simulink model "Model_TranslationEngine64"  (R2022b)
settings: Solver=FixedStepDiscrete  StartTime=0.0  StopTime=5  RelTol=1e-3  EnableMultiTasking=on
InitFcn:
  | % Initialize model
  | ModelSettings=BTConfig.GetModelSettings();
  | 
  | ModelSettings.Validate();
  | 
  | ModelInit;
  | 
  | 
  | % load library data
  | GainLibrary_data;
  | % Load saved values from partition process
  | CapturedConstMask.LoadMapFromFile(bdroot)
StartFcn:
  | % make sure all the simulated RTC requests are found
  | %RTC_SIM_OBJ.ValidateREQs();
undefined symbols (not defined in the file or in its folder): AA, BPLP, Column, NumHFRefBPF, NumHFRefLPF, NumMusicChannels, Row, VolumeMuteConfig
libraries: TuneVar x925, TOP x490, FeaturePath x111, CapturedConstLib x52
(part 4 of 34)

== system Model_TranslationEngine64/NEAR/Near1p1/VolumeMute/VolMuteCh1 ==
  Ann1NonEntGainCalc : Subsystem  mask(Blocklib NonEntGainCalc){Config=Config.Ann1NonEntGainCalc, FeatureName=Ann1NonEntGainCalc}
      mask prompts: Config "NonEntGainCalcConfig"; FeatureName "Feature path name:"
      mask init:
      | blkh=gcbh;
      | Config=BTConfig.Assert(blkh,Config);
      | 
      | Config.Validate();
      | BTConfig.InitSetFeatureIfPresent(blkh,'FeatureName');
      | 
      | % Flatten for MFB is not needed due to mask on MFB. Nice.
      mask Callback Config: BTConfig.CallbackHideIfPresent(gcbh,{'FeatureName'});
      mask TypeOptions FeatureName: FeaturePath/FeatureName
      mask DialogControl ParameterGroupVar2 Prompt: OverRides
  Ann1NonEntVncApplied : Subsystem  mask(Blocklib NonEntVncApplied){Config=Config.Ann1NonEntVncApplied, FeatureName=Ann1NonEntVncApplied}
      mask prompts: Config "NonEntVncAppliedConfig"; FeatureName "Feature path name:"
      mask init:
      | blkh=gcbh;
      | Config=BTConfig.Assert(blkh,Config);
      | Config.Validate();
      | BTConfig.InitSetFeatureIfPresent(blkh,'FeatureName');
      mask Callback Config: BTConfig.CallbackHideIfPresent(gcbh,{'FeatureName'});
      mask TypeOptions FeatureName: FeaturePath/FeatureName
  FeaturePath : FeaturePath/FeaturePath  FeatureName=Ann1  IsGroup=off  GroupNumber=-1  IsModule=off  TriggerInit=[270 -291 385 -184]
      settings: SourceProductName=Bose Talaria
  Mute : Subsystem  mask(Blocklib Mute){Config=Config.Ann1Mute, FeatureName=Ann1Mute}
      mask prompts: Config "MuteConfig"; FeatureName "Feature path name:"
      mask help: This block offers a simple mute feature using rgainy block. Set initial mute state for system cold start and a feature path name as desired. There are no tunable components, but runtime control is included.
      mask init:
      | blkh=gcbh;
      | Config=BTConfig.Assert(blkh,Config);
      | BTConfig.InitSetFeatureIfPresent(blkh,'FeatureName');
      | Config.Validate();
      mask Help:
      | This block offers a simple mute feature using rgainy block. The initial mute status of the block can be set through the mask.
      | 
      | RTC CONTROL:
      | Run time control is available to dynamically mute the audio. The mute status can be provided ('1' to mute audio), along with a ramp time and rate (rate gets precedence).
      | RTC_SIM_OBJ.AddREQ( 'MuteSet', 0.6, [0005,  <mute_status>, <ramp_db_per_second>, <ramp_time>]);
      | E.g., RTC_SIM_OBJ.AddREQ( 'MuteSet', 0.7, [0002, 1, 0, 50]);
      mask Callback Config: BTConfig.CallbackHideIfPresent(gcbh,{'FeatureName'});
      mask TypeOptions FeatureName: MuteControl/FeatureName
      mask Display:
      | [path,w,h] = IconMuteMask();
      | 
      | % work in pixels since the icon does not scale
      | pos = get(gcbh,'position');
      | bw = pos(3) - pos(1);
      | bh = pos(4) - pos(2);
      | 
      | % Draw centered icon
      | xAdj = bw/2 - w/2;
      | yAdj = bh/2 - h/2;
      | for i=1:length(path)
      |     if (path(i).rgb(1) >= 0)
      |         patch(path(i).x+xAdj, path(i).y+yAdj, path(i).rgb);
      |     end
      |     if (path(i).stroke(1) >= 0)
      |         plot(path(i).x+xAdj, path(i).y+yAdj);
      |     end
      | end
      | 
      | % Display some text
      | text(bw/2, 2,FeatureName, ...
      |     'horizontalAlignment','center', ...
      |     'VerticalAlignment','bottom');
  Volume : Subsystem  mask(Blocklib AnnVolume){FeatureName=Ann1Volume, Config=Config.Ann1Volume, TriggerInit=[50 25 130 85]}
      mask prompts: FeatureName "Feature path name:"; Config "AnnVolumeConfig"; TriggerInit "Hidden: MoveFcn redraw"
      mask help: This volume signal block includes receipt of volume level (via RTC) as well as tuning variables to calibrate a gain table that maps 8-bit integer volume index (from RTC) to float decibels.
      mask init:
      | blkh=gcbh;
      | Config=BTConfig.Assert(blkh,Config);
      | BTConfig.InitSetFeatureIfPresent(blkh,'FeatureName');
      | Config.Validate();
      settings: MoveFcn=VolumeMask.CB_TriggerInit(gcbh);
      mask TypeOptions FeatureName: FeaturePath/FeatureName
      mask Callback Config: BTConfig.CallbackHideIfPresent(gcbh,{'FeatureName'});
      mask Callback TriggerInit: VolumeMask.CB_TriggerInit(gcbh);
      mask Display:
      | [path,w,h] = IconVolumeMask();
      | 
      | % work in pixels since the icon does not scale
      | pos = get(gcbh,'position');
      | bw = pos(3) - pos(1);
      | bh = pos(4) - pos(2);
      | 
      | % Draw centered icon
      | xAdj = bw/2 - w/2;
      | yAdj = bh/2 - h/2;
      | for i=1:length(path)
      |     if (path(i).rgb(1) >= 0)
      |         patch(path(i).x+xAdj, path(i).y+yAdj, path(i).rgb);
      |     end
      |     if (path(i).stroke(1) >= 0)
      |         plot(path(i).x+xAdj, path(i).y+yAdj);
      |     end
      | end
      | 
      | % Display some text
      | text(bw/2, bh/2,FeatureName, ...
      |     'horizontalAlignment','center', ...
      |     'VerticalAlignment','middle');

== system Model_TranslationEngine64/NEAR/Near1p1/VolumeMute/VolMuteCh2 ==
  Ann2NonEntGainCalc : Subsystem  mask(Blocklib NonEntGainCalc){Config=Config.Ann2NonEntGainCalc, FeatureName=Ann2NonEntGainCalc}
      mask prompts: Config "NonEntGainCalcConfig"; FeatureName "Feature path name:"
      mask init:
      | blkh=gcbh;
      | Config=BTConfig.Assert(blkh,Config);
      | 
      | Config.Validate();
      | BTConfig.InitSetFeatureIfPresent(blkh,'FeatureName');
      | 
      | % Flatten for MFB is not needed due to mask on MFB. Nice.
      mask Callback Config: BTConfig.CallbackHideIfPresent(gcbh,{'FeatureName'});
      mask TypeOptions FeatureName: FeaturePath/FeatureName
      mask DialogControl ParameterGroupVar2 Prompt: OverRides
  Ann2NonEntVncApplied : Subsystem  mask(Blocklib NonEntVncApplied){Config=Config.Ann2NonEntVncApplied, FeatureName=Ann2NonEntVncApplied}
      mask prompts: Config "NonEntVncAppliedConfig"; FeatureName "Feature path name:"
      mask init:
      | blkh=gcbh;
      | Config=BTConfig.Assert(blkh,Config);
      | Config.Validate();
      | BTConfig.InitSetFeatureIfPresent(blkh,'FeatureName');
      mask Callback Config: BTConfig.CallbackHideIfPresent(gcbh,{'FeatureName'});
      mask TypeOptions FeatureName: FeaturePath/FeatureName
  FeaturePath : FeaturePath/FeaturePath  FeatureName=Ann2  IsGroup=off  GroupNumber=-1  IsModule=off  TriggerInit=[60 -206 175 -99]
      settings: SourceProductName=Bose Talaria
  Mute : Subsystem  mask(Blocklib Mute){Config=Config.Ann2Mute, FeatureName=Ann2Mute}
      mask prompts: Config "MuteConfig"; FeatureName "Feature path name:"
      mask help: This block offers a simple mute feature using rgainy block. Set initial mute state for system cold start and a feature path name as desired. There are no tunable components, but runtime control is included.
      mask init:
      | blkh=gcbh;
      | Config=BTConfig.Assert(blkh,Config);
      | BTConfig.InitSetFeatureIfPresent(blkh,'FeatureName');
      | Config.Validate();
      mask Help:
      | This block offers a simple mute feature using rgainy block. The initial mute status of the block can be set through the mask.
      | 
      | RTC CONTROL:
      | Run time control is available to dynamically mute the audio. The mute status can be provided ('1' to mute audio), along with a ramp time and rate (rate gets precedence).
      | RTC_SIM_OBJ.AddREQ( 'MuteSet', 0.6, [0005,  <mute_status>, <ramp_db_per_second>, <ramp_time>]);
      | E.g., RTC_SIM_OBJ.AddREQ( 'MuteSet', 0.7, [0002, 1, 0, 50]);
      mask Callback Config: BTConfig.CallbackHideIfPresent(gcbh,{'FeatureName'});
      mask TypeOptions FeatureName: MuteControl/FeatureName
      mask Display:
      | [path,w,h] = IconMuteMask();
      | 
      | % work in pixels since the icon does not scale
      | pos = get(gcbh,'position');
      | bw = pos(3) - pos(1);
      | bh = pos(4) - pos(2);
      | 
      | % Draw centered icon
      | xAdj = bw/2 - w/2;
      | yAdj = bh/2 - h/2;
      | for i=1:length(path)
      |     if (path(i).rgb(1) >= 0)
      |         patch(path(i).x+xAdj, path(i).y+yAdj, path(i).rgb);
      |     end
      |     if (path(i).stroke(1) >= 0)
      |         plot(path(i).x+xAdj, path(i).y+yAdj);
      |     end
      | end
      | 
      | % Display some text
      | text(bw/2, 2,FeatureName, ...
      |     'horizontalAlignment','center', ...
      |     'VerticalAlignment','bottom');
  Volume : Subsystem  mask(Blocklib AnnVolume){FeatureName=Ann2Volume, Config=Config.Ann2Volume, TriggerInit=[0 -25 80 35]}
      mask prompts: FeatureName "Feature path name:"; Config "AnnVolumeConfig"; TriggerInit "Hidden: MoveFcn redraw"
      mask help: This volume signal block includes receipt of volume level (via RTC) as well as tuning variables to calibrate a gain table that maps 8-bit integer volume index (from RTC) to float decibels.
      mask init:
      | blkh=gcbh;
      | Config=BTConfig.Assert(blkh,Config);
      | BTConfig.InitSetFeatureIfPresent(blkh,'FeatureName');
      | Config.Validate();
      settings: MoveFcn=VolumeMask.CB_TriggerInit(gcbh);
      mask TypeOptions FeatureName: FeaturePath/FeatureName
      mask Callback Config: BTConfig.CallbackHideIfPresent(gcbh,{'FeatureName'});
      mask Callback TriggerInit: VolumeMask.CB_TriggerInit(gcbh);
      mask Display:
      | [path,w,h] = IconVolumeMask();
      | 
      | % work in pixels since the icon does not scale
      | pos = get(gcbh,'position');
      | bw = pos(3) - pos(1);
      | bh = pos(4) - pos(2);
      | 
      | % Draw centered icon
      | xAdj = bw/2 - w/2;
      | yAdj = bh/2 - h/2;
      | for i=1:length(path)
      |     if (path(i).rgb(1) >= 0)
      |         patch(path(i).x+xAdj, path(i).y+yAdj, path(i).rgb);
      |     end
      |     if (path(i).stroke(1) >= 0)
      |         plot(path(i).x+xAdj, path(i).y+yAdj);
      |     end
      | end
      | 
      | % Display some text
      | text(bw/2, bh/2,FeatureName, ...
      |     'horizontalAlignment','center', ...
      |     'VerticalAlignment','middle');

== system Model_TranslationEngine64/NEAR/Near1p1/VolumeMute/VolMuteCh3 ==
  Ann3NonEntGainCalc : Subsystem  mask(Blocklib NonEntGainCalc){Config=Config.Ann3NonEntGainCalc, FeatureName=Ann3NonEntGainCalc}
      mask prompts: Config "NonEntGainCalcConfig"; FeatureName "Feature path name:"
      mask init:
      | blkh=gcbh;
      | Config=BTConfig.Assert(blkh,Config);
      | 
      | Config.Validate();
      | BTConfig.InitSetFeatureIfPresent(blkh,'FeatureName');
      | 
      | % Flatten for MFB is not needed due to mask on MFB. Nice.
      mask Callback Config: BTConfig.CallbackHideIfPresent(gcbh,{'FeatureName'});
      mask TypeOptions FeatureName: FeaturePath/FeatureName
      mask DialogControl ParameterGroupVar2 Prompt: OverRides
  Ann3NonEntVncApplied : Subsystem  mask(Blocklib NonEntVncApplied){Config=Config.Ann3NonEntVncApplied, FeatureName=Ann3NonEntVncApplied}
      mask prompts: Config "NonEntVncAppliedConfig"; FeatureName "Feature path name:"
      mask init:
      | blkh=gcbh;
      | Config=BTConfig.Assert(blkh,Config);
      | Config.Validate();
      | BTConfig.InitSetFeatureIfPresent(blkh,'FeatureName');
      mask Callback Config: BTConfig.CallbackHideIfPresent(gcbh,{'FeatureName'});
      mask TypeOptions FeatureName: FeaturePath/FeatureName
  FeaturePath : FeaturePath/FeaturePath  FeatureName=Ann3  IsGroup=off  GroupNumber=-1  IsModule=off  TriggerInit=[265 -336 380 -229]
      settings: SourceProductName=Bose Talaria
  Mute : Subsystem  mask(Blocklib Mute){Config=Config.Ann3Mute, FeatureName=Ann3Mute}
      mask prompts: Config "MuteConfig"; FeatureName "Feature path name:"
      mask help: This block offers a simple mute feature using rgainy block. Set initial mute state for system cold start and a feature path name as desired. There are no tunable components, but runtime control is included.
      mask init:
      | blkh=gcbh;
      | Config=BTConfig.Assert(blkh,Config);
      | BTConfig.InitSetFeatureIfPresent(blkh,'FeatureName');
      | Config.Validate();
      mask Help:
      | This block offers a simple mute feature using rgainy block. The initial mute status of the block can be set through the mask.
      | 
      | RTC CONTROL:
      | Run time control is available to dynamically mute the audio. The mute status can be provided ('1' to mute audio), along with a ramp time and rate (rate gets precedence).
      | RTC_SIM_OBJ.AddREQ( 'MuteSet', 0.6, [0005,  <mute_status>, <ramp_db_per_second>, <ramp_time>]);
      | E.g., RTC_SIM_OBJ.AddREQ( 'MuteSet', 0.7, [0002, 1, 0, 50]);
      mask Callback Config: BTConfig.CallbackHideIfPresent(gcbh,{'FeatureName'});
      mask TypeOptions FeatureName: MuteControl/FeatureName
      mask Display:
      | [path,w,h] = IconMuteMask();
      | 
      | % work in pixels since the icon does not scale
      | pos = get(gcbh,'position');
      | bw = pos(3) - pos(1);
      | bh = pos(4) - pos(2);
      | 
      | % Draw centered icon
      | xAdj = bw/2 - w/2;
      | yAdj = bh/2 - h/2;
      | for i=1:length(path)
      |     if (path(i).rgb(1) >= 0)
      |         patch(path(i).x+xAdj, path(i).y+yAdj, path(i).rgb);
      |     end
      |     if (path(i).stroke(1) >= 0)
      |         plot(path(i).x+xAdj, path(i).y+yAdj);
      |     end
      | end
      | 
      | % Display some text
      | text(bw/2, 2,FeatureName, ...
      |     'horizontalAlignment','center', ...
      |     'VerticalAlignment','bottom');
  Volume : Subsystem  mask(Blocklib AnnVolume){FeatureName=Ann3Volume, Config=Config.Ann3Volume, TriggerInit=[815 415 895 475]}
      mask prompts: FeatureName "Feature path name:"; Config "AnnVolumeConfig"; TriggerInit "Hidden: MoveFcn redraw"
      mask help: This volume signal block includes receipt of volume level (via RTC) as well as tuning variables to calibrate a gain table that maps 8-bit integer volume index (from RTC) to float decibels.
      mask init:
      | blkh=gcbh;
      | Config=BTConfig.Assert(blkh,Config);
      | BTConfig.InitSetFeatureIfPresent(blkh,'FeatureName');
      | Config.Validate();
      settings: MoveFcn=VolumeMask.CB_TriggerInit(gcbh);
      mask TypeOptions FeatureName: FeaturePath/FeatureName
      mask Callback Config: BTConfig.CallbackHideIfPresent(gcbh,{'FeatureName'});
      mask Callback TriggerInit: VolumeMask.CB_TriggerInit(gcbh);
      mask Display:
      | [path,w,h] = IconVolumeMask();
      | 
      | % work in pixels since the icon does not scale
      | pos = get(gcbh,'position');
      | bw = pos(3) - pos(1);
      | bh = pos(4) - pos(2);
      | 
      | % Draw centered icon
      | xAdj = bw/2 - w/2;
      | yAdj = bh/2 - h/2;
      | for i=1:length(path)
      |     if (path(i).rgb(1) >= 0)
      |         patch(path(i).x+xAdj, path(i).y+yAdj, path(i).rgb);
      |     end
      |     if (path(i).stroke(1) >= 0)
      |         plot(path(i).x+xAdj, path(i).y+yAdj);
      |     end
      | end
      | 
      | % Display some text
      | text(bw/2, bh/2,FeatureName, ...
      |     'horizontalAlignment','center', ...
      |     'VerticalAlignment','middle');

== system Model_TranslationEngine64/NEAR/Near1p1/VolumeMute/VolMuteCh4 ==
  Ann4NonEntGainCalc : Subsystem  mask(Blocklib NonEntGainCalc){Config=Config.Ann4NonEntGainCalc, FeatureName=Ann4NonEntGainCalc}
      mask prompts: Config "NonEntGainCalcConfig"; FeatureName "Feature path name:"
      mask init:
      | blkh=gcbh;
      | Config=BTConfig.Assert(blkh,Config);
      | 
      | Config.Validate();
      | BTConfig.InitSetFeatureIfPresent(blkh,'FeatureName');
      | 
      | % Flatten for MFB is not needed due to mask on MFB. Nice.
      mask Callback Config: BTConfig.CallbackHideIfPresent(gcbh,{'FeatureName'});
      mask TypeOptions FeatureName: FeaturePath/FeatureName
      mask DialogControl ParameterGroupVar2 Prompt: OverRides
  Ann4NonEntVncApplied : Subsystem  mask(Blocklib NonEntVncApplied){Config=Config.Ann4NonEntVncApplied, FeatureName=Ann4NonEntVncApplied}
      mask prompts: Config "NonEntVncAppliedConfig"; FeatureName "Feature path name:"
      mask init:
      | blkh=gcbh;
      | Config=BTConfig.Assert(blkh,Config);
      | Config.Validate();
      | BTConfig.InitSetFeatureIfPresent(blkh,'FeatureName');
      mask Callback Config: BTConfig.CallbackHideIfPresent(gcbh,{'FeatureName'});
      mask TypeOptions FeatureName: FeaturePath/FeatureName
  FeaturePath : FeaturePath/FeaturePath  FeatureName=Ann4  IsGroup=off  GroupNumber=-1  IsModule=off  TriggerInit=[235 -186 350 -79]
      settings: SourceProductName=Bose Talaria
  Mute : Subsystem  mask(Blocklib Mute){Config=Config.Ann4Mute, FeatureName=Ann4Mute}
      mask prompts: Config "MuteConfig"; FeatureName "Feature path name:"
      mask help: This block offers a simple mute feature using rgainy block. Set initial mute state for system cold start and a feature path name as desired. There are no tunable components, but runtime control is included.
      mask init:
      | blkh=gcbh;
      | Config=BTConfig.Assert(blkh,Config);
      | BTConfig.InitSetFeatureIfPresent(blkh,'FeatureName');
      | Config.Validate();
      mask Help:
      | This block offers a simple mute feature using rgainy block. The initial mute status of the block can be set through the mask.
      | 
      | RTC CONTROL:
      | Run time control is available to dynamically mute the audio. The mute status can be provided ('1' to mute audio), along with a ramp time and rate (rate gets precedence).
      | RTC_SIM_OBJ.AddREQ( 'MuteSet', 0.6, [0005,  <mute_status>, <ramp_db_per_second>, <ramp_time>]);
      | E.g., RTC_SIM_OBJ.AddREQ( 'MuteSet', 0.7, [0002, 1, 0, 50]);
      mask Callback Config: BTConfig.CallbackHideIfPresent(gcbh,{'FeatureName'});
      mask TypeOptions FeatureName: MuteControl/FeatureName
      mask Display:
      | [path,w,h] = IconMuteMask();
      | 
      | % work in pixels since the icon does not scale
      | pos = get(gcbh,'position');
      | bw = pos(3) - pos(1);
      | bh = pos(4) - pos(2);
      | 
      | % Draw centered icon
      | xAdj = bw/2 - w/2;
      | yAdj = bh/2 - h/2;
      | for i=1:length(path)
      |     if (path(i).rgb(1) >= 0)
      |         patch(path(i).x+xAdj, path(i).y+yAdj, path(i).rgb);
      |     end
      |     if (path(i).stroke(1) >= 0)
      |         plot(path(i).x+xAdj, path(i).y+yAdj);
      |     end
      | end
      | 
      | % Display some text
      | text(bw/2, 2,FeatureName, ...
      |     'horizontalAlignment','center', ...
      |     'VerticalAlignment','bottom');
  Volume : Subsystem  mask(Blocklib AnnVolume){FeatureName=Ann4Volume, Config=Config.Ann4Volume, TriggerInit=[20 5 100 65]}
      mask prompts: FeatureName "Feature path name:"; Config "AnnVolumeConfig"; TriggerInit "Hidden: MoveFcn redraw"
      mask help: This volume signal block includes receipt of volume level (via RTC) as well as tuning variables to calibrate a gain table that maps 8-bit integer volume index (from RTC) to float decibels.
      mask init:
      | blkh=gcbh;
      | Config=BTConfig.Assert(blkh,Config);
      | BTConfig.InitSetFeatureIfPresent(blkh,'FeatureName');
      | Config.Validate();
      settings: MoveFcn=VolumeMask.CB_TriggerInit(gcbh);
      mask TypeOptions FeatureName: FeaturePath/FeatureName
      mask Callback Config: BTConfig.CallbackHideIfPresent(gcbh,{'FeatureName'});
      mask Callback TriggerInit: VolumeMask.CB_TriggerInit(gcbh);
      mask Display:
      | [path,w,h] = IconVolumeMask();
      | 
      | % work in pixels since the icon does not scale
      | pos = get(gcbh,'position');
      | bw = pos(3) - pos(1);
      | bh = pos(4) - pos(2);
      | 
      | % Draw centered icon
      | xAdj = bw/2 - w/2;
      | yAdj = bh/2 - h/2;
      | for i=1:length(path)
      |     if (path(i).rgb(1) >= 0)
      |         patch(path(i).x+xAdj, path(i).y+yAdj, path(i).rgb);
      |     end
      |     if (path(i).stroke(1) >= 0)
      |         plot(path(i).x+xAdj, path(i).y+yAdj);
      |     end
      | end
      | 
      | % Display some text
      | text(bw/2, bh/2,FeatureName, ...
      |     'horizontalAlignment','center', ...
      |     'VerticalAlignment','middle');

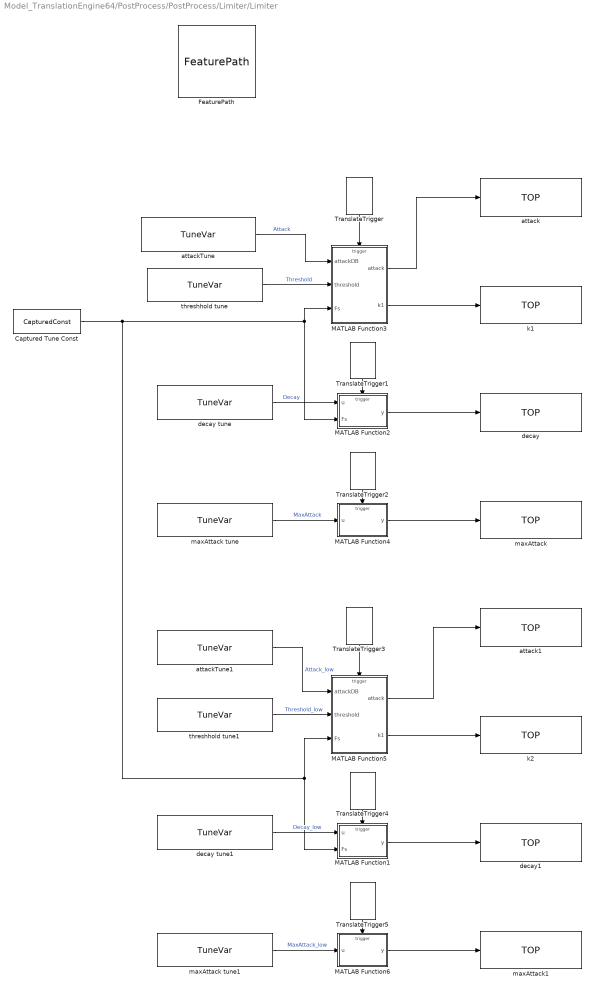
== system Model_TranslationEngine64/PostProcess/PostProcess/Limiter/Limiter ==
  Captured Tune Const : CapturedConstLib/CapturedConst  TriggerInit=[-235 487 -135 523]  Role=Automatic
      settings: SourceProductName=Bose Talaria
  FeaturePath : FeaturePath/FeaturePath  FeatureName=Limiter  IsGroup=off  GroupNumber=-1  IsModule=off  TriggerInit=[10 64 125 171]
      settings: SourceProductName=Bose Talaria
  MATLAB Function1 : MATLAB Function  TreatAsAtomicUnit=on
  MATLAB Function2 : MATLAB Function  TreatAsAtomicUnit=on
  MATLAB Function3 : MATLAB Function  TreatAsAtomicUnit=on
  MATLAB Function4 : MATLAB Function  TreatAsAtomicUnit=on
  MATLAB Function5 : MATLAB Function  TreatAsAtomicUnit=on
  MATLAB Function6 : MATLAB Function  TreatAsAtomicUnit=on
  TranslateTrigger : TuneVar/TranslateTrigger  TriggerInit=[261 290 299 345]
      settings: SourceProductName=Bose Talaria
  TranslateTrigger1 : TuneVar/TranslateTrigger  TriggerInit=[266 535 304 590]
      settings: SourceProductName=Bose Talaria
  TranslateTrigger2 : TuneVar/TranslateTrigger  TriggerInit=[266 700 304 755]
      settings: SourceProductName=Bose Talaria
  TranslateTrigger3 : TuneVar/TranslateTrigger  TriggerInit=[261 930 299 985]
      settings: SourceProductName=Bose Talaria
  TranslateTrigger4 : TuneVar/TranslateTrigger  TriggerInit=[266 1175 304 1230]
      settings: SourceProductName=Bose Talaria
  TranslateTrigger5 : TuneVar/TranslateTrigger  TriggerInit=[266 1340 304 1395]
      settings: SourceProductName=Bose Talaria
  attack : TOP/TOP  TriggerInit=[460 292 610 348]  TopName=attack  DataTypeOut=single  BankNumber=0  PreOverlay=false  PostOverlay=false  Role=Automatic
      settings: SourceProductName=Bose Talaria
  attack1 : TOP/TOP  TriggerInit=[460 932 610 988]  TopName=attack_low  DataTypeOut=single  BankNumber=0  PreOverlay=false  PostOverlay=false  Role=Automatic
      settings: SourceProductName=Bose Talaria
  attackTune : TuneVar/TuneVar  TuneName=Attack  SpecifyMaxSize=off  VariableDim=2 (Column)  MaxSize=[1 16]  TunabilityNumber=1  MinValue=[]  MaxValue=[]  TriggerInit=[-45 350 125 400]  MaskValue=Config.DefaultAttackDb
      settings: SourceProductName=Bose Talaria
  attackTune1 : TuneVar/TuneVar  TuneName=Attack_low  SpecifyMaxSize=off  VariableDim=2 (Column)  MaxSize=[1 1]  TunabilityNumber=1  MinValue=[]  MaxValue=[]  TriggerInit=[-20 965 150 1015]  MaskValue=Config.DefaultAttackLowDb
      settings: SourceProductName=Bose Talaria
  decay : TOP/TOP  TriggerInit=[460 612 610 668]  TopName=decay  DataTypeOut=single  BankNumber=0  PreOverlay=false  PostOverlay=false  Role=Automatic
      settings: SourceProductName=Bose Talaria
  decay tune : TuneVar/TuneVar  TuneName=Decay  SpecifyMaxSize=off  VariableDim=2 (Column)  MaxSize=[1 1]  TunabilityNumber=1  MinValue=[]  MaxValue=[]  TriggerInit=[-20 600 150 650]  MaskValue=Config.DefaultDecayDB
      settings: SourceProductName=Bose Talaria
  decay tune1 : TuneVar/TuneVar  TuneName=Decay_low  SpecifyMaxSize=off  VariableDim=2 (Column)  MaxSize=[1 1]  TunabilityNumber=1  MinValue=[]  MaxValue=[]  TriggerInit=[-20 1240 150 1290]  MaskValue=Config.DefaultDecayLowDb
      settings: SourceProductName=Bose Talaria
  decay1 : TOP/TOP  TriggerInit=[460 1252 610 1308]  TopName=decay_low  DataTypeOut=single  BankNumber=0  PreOverlay=false  PostOverlay=false  Role=Automatic
      settings: SourceProductName=Bose Talaria
  k1 : TOP/TOP  TriggerInit=[460 452 610 508]  TopName=k1  DataTypeOut=single  BankNumber=0  PreOverlay=false  PostOverlay=false  Role=Automatic
      settings: SourceProductName=Bose Talaria
  k2 : TOP/TOP  TriggerInit=[460 1092 610 1148]  TopName=k1_low  DataTypeOut=single  BankNumber=0  PreOverlay=false  PostOverlay=false  Role=Automatic
      settings: SourceProductName=Bose Talaria
  maxAttack : TOP/TOP  TriggerInit=[460 772 610 828]  TopName=maxAttack  DataTypeOut=single  BankNumber=0  PreOverlay=false  PostOverlay=false  Role=Automatic
      settings: SourceProductName=Bose Talaria
  maxAttack tune : TuneVar/TuneVar  TuneName=MaxAttack  SpecifyMaxSize=off  VariableDim=2 (Column)  MaxSize=[1 1]  TunabilityNumber=1  MinValue=[]  MaxValue=[]  TriggerInit=[-20 775 150 825]  MaskValue=Config.DefaultMaxAttackDb
      settings: SourceProductName=Bose Talaria
  maxAttack tune1 : TuneVar/TuneVar  TuneName=MaxAttack_low  SpecifyMaxSize=off  VariableDim=2 (Column)  MaxSize=[1 1]  TunabilityNumber=1  MinValue=[]  MaxValue=[]  TriggerInit=[-20 1415 150 1465]  MaskValue=Config.DefaultMaxAttackLowDb
      settings: SourceProductName=Bose Talaria
  maxAttack1 : TOP/TOP  TriggerInit=[460 1412 610 1468]  TopName=maxAttack_low  DataTypeOut=single  BankNumber=0  PreOverlay=false  PostOverlay=false  Role=Automatic
      settings: SourceProductName=Bose Talaria
  threshhold tune : TuneVar/TuneVar  TuneName=Threshold  SpecifyMaxSize=off  VariableDim=2 (Column)  MaxSize=[1 16]  TunabilityNumber=1  MinValue=[]  MaxValue=[]  TriggerInit=[-35 425 135 475]  MaskValue=Config.DefaultThreshold
      settings: SourceProductName=Bose Talaria
  threshhold tune1 : TuneVar/TuneVar  TuneName=Threshold_low  SpecifyMaxSize=off  VariableDim=2 (Column)  MaxSize=[1 1]  TunabilityNumber=1  MinValue=[]  MaxValue=[]  TriggerInit=[-20 1065 150 1115]  MaskValue=Config.DefaultThresholdLow
      settings: SourceProductName=Bose Talaria
  wires:
  TranslateTrigger4/1 -> MATLAB Function1/Trigger
  maxAttack tune1/1 -> MATLAB Function6/1(u)  "MaxAttack_low"
  TranslateTrigger3/1 -> MATLAB Function5/Trigger
  MATLAB Function5/2(k1) -> k2/1
  threshhold tune1/1 -> MATLAB Function5/2(threshold)  "Threshold_low"
  attackTune1/1 -> MATLAB Function5/1(attackDB)  "Attack_low"
  decay tune1/1 -> MATLAB Function1/1(u)  "Decay_low"
  MATLAB Function1/1(y) -> decay1/1
  Captured Tune Const/1 -> MATLAB Function1/2(Fs), MATLAB Function5/3(Fs), MATLAB Function2/2(Fs), MATLAB Function3/3(Fs)
  TranslateTrigger5/1 -> MATLAB Function6/Trigger
  MATLAB Function6/1(y) -> maxAttack1/1
  MATLAB Function5/1(attack) -> attack1/1
  MATLAB Function3/1(attack) -> attack/1
  MATLAB Function4/1(y) -> maxAttack/1
  TranslateTrigger2/1 -> MATLAB Function4/Trigger
  maxAttack tune/1 -> MATLAB Function4/1(u)  "MaxAttack"
  MATLAB Function3/2(k1) -> k1/1
  TranslateTrigger/1 -> MATLAB Function3/Trigger
  threshhold tune/1 -> MATLAB Function3/2(threshold)  "Threshold"
  MATLAB Function2/1(y) -> decay/1
  TranslateTrigger1/1 -> MATLAB Function2/Trigger
  decay tune/1 -> MATLAB Function2/1(u)  "Decay"
  attackTune/1 -> MATLAB Function3/1(attackDB)  "Attack"

== system Model_TranslationEngine64/PostProcess/PostProcess/Mute/Mute ==
  MuteControl : Subsystem  mask(Blocklib MuteControl){Config=Config, FeatureName=Mute}
      mask prompts: Config "MuteControlConfig"; FeatureName "Mask feature name:"
      mask help: This component is to be used in conjunction with 1 or more instances of the MuteRamper block. There is no mask for this component. It provides the control layer for Mute processing via an RTC and tune variable, muteControlRampTime.
      mask init:
      | blkh=gcbh;
      | Config=BTConfig.Assert(blkh,Config);
      | BTConfig.InitSetFeatureIfPresent(blkh,'FeatureName');
      | Config.Validate();
      | 
      | % Set boundary conditions
      | rampRateBounds = [5,50000];
      | rampTimeBounds = [1,3000];
      mask Help: If this control block is being used in a "multi-instance" manner, i.e. it is contorlling two or more MuteRamper blocks, there is an additional step that must be done. The developer must add a function-triggered subsytem containing an AND logic gate, which will combine the notification completion signals of the multiple ramper instances. The output of this subsytem must then feed the NTF_done input of the MuteControl block.
      mask Callback Config: BTConfig.CallbackHideIfPresent(gcbh,{'FeatureName'});
      mask TypeOptions FeatureName: FeaturePath/FeatureName

== system Model_TranslationEngine64/PostProcess/PostProcess/PostLimiterEQ/PoolIirTunableWithReset ==
  CapturedTuneConst : CapturedConstLib/CapturedConst  TriggerInit=[-600 302 -500 338]  Role=Automatic
      settings: SourceProductName=Bose Talaria
  FeaturePath : FeaturePath/FeaturePath  FeatureName=PostLimiterEq  IsGroup=off  GroupNumber=-1  IsModule=off  TriggerInit=[-750 -81 -635 26]
      settings: SourceProductName=Bose Talaria
  TOP : TOP/TOP  TriggerInit=[-145 187 5 243]  TopName=PooliirNumStages  DataTypeOut=uint32  BankNumber=0  PreOverlay=false  PostOverlay=Config.VariantObj.PostOverlayRequired  Role=Automatic
      settings: SourceProductName=Bose Talaria
  TOP1 : TOP/TOP  TriggerInit=[-140 277 10 333]  TopName=pooliirCoeffs  DataTypeOut=single  BankNumber=0  PreOverlay=false  PostOverlay=Config.VariantObj.PostOverlayRequired  Role=Automatic
      settings: SourceProductName=Bose Talaria
  TranslateTrigger : TuneVar/TranslateTrigger  TriggerInit=[-339 35 -301 90]
      settings: SourceProductName=Bose Talaria
  Translation : MATLAB Function  TreatAsAtomicUnit=on  mask{MaxNumStages=Config.MaxNumStages, VariantUint8=Config.Variant.Uint8Str}
      mask prompts: VariantUint8 "Variant"
  Tune Variable1 : TuneVar/TuneVar  TuneName=numStages  SpecifyMaxSize=off  VariableDim=1 (Row)  MaxSize=[1 1]  TunabilityNumber=1  MinValue=[]  MaxValue=[]  TriggerInit=[-750 235 -580 285]  MaskValue=Config.TuneDefaults.NumStages
      settings: SourceProductName=Bose Talaria
  Tune Variable2 : TuneVar/TuneVar  TuneName=sosCoefficients  SpecifyMaxSize=on  VariableDim=1 (Row)  MaxSize=[Config.MaxNumStages 6]  TunabilityNumber=1  MinValue=[]  MaxValue=[]  TriggerInit=[-750 175 -580 225]  MaskValue=Config.TuneDefaults.SosCoefficients
      settings: SourceProductName=Bose Talaria
  wires:
  CapturedTuneConst/1 -> Translation/3(NumChannels)
  Tune Variable1/1 -> Translation/2(NumStages)  "numStages"
  Translation/1(PoolNumStages) -> TOP/1
  Translation/2(PoolCoeffs) -> TOP1/1
  Tune Variable2/1 -> Translation/1(RawSOS)  "sosCoefficients"
  TranslateTrigger/1 -> Translation/Trigger

== system Model_TranslationEngine64/PostProcess/PostProcess/Soft Clipper/SoftClipper ==
  FeaturePath : FeaturePath/FeaturePath  FeatureName=SoftClipper  IsGroup=off  GroupNumber=-1  IsModule=off  TriggerInit=[-80 -61 25 36]
      settings: SourceProductName=Bose Talaria
  TranslateTrigger : TuneVar/TranslateTrigger  TriggerInit=[341 -20 379 35]
      settings: SourceProductName=Bose Talaria
  TranslateTrigger1 : TuneVar/TranslateTrigger  TriggerInit=[341 350 379 405]
      settings: SourceProductName=Bose Talaria
  p2 TOP : TOP/TOP  TriggerInit=[525 247 675 303]  TopName=p2  DataTypeOut=single  BankNumber=0  PreOverlay=false  PostOverlay=false  Role=Automatic
      settings: SourceProductName=Bose Talaria
  p2 TOP1 : TOP/TOP  TriggerInit=[525 587 675 643]  TopName=p2_low  DataTypeOut=single  BankNumber=0  PreOverlay=false  PostOverlay=false  Role=Automatic
      settings: SourceProductName=Bose Talaria
  translation : MATLAB Function  TreatAsAtomicUnit=on
  translation1 : MATLAB Function  TreatAsAtomicUnit=on
  xmax TOP : TOP/TOP  TriggerInit=[525 172 675 228]  TopName=xmax  DataTypeOut=single  BankNumber=0  PreOverlay=false  PostOverlay=false  Role=Automatic
      settings: SourceProductName=Bose Talaria
  xmax TOP1 : TOP/TOP  TriggerInit=[525 512 675 568]  TopName=xmax_low  DataTypeOut=single  BankNumber=0  PreOverlay=false  PostOverlay=false  Role=Automatic
      settings: SourceProductName=Bose Talaria
  xmin TOP : TOP/TOP  TriggerInit=[525 97 675 153]  TopName=xmin  DataTypeOut=single  BankNumber=0  PreOverlay=false  PostOverlay=false  Role=Automatic
      settings: SourceProductName=Bose Talaria
  xmin TOP1 : TOP/TOP  TriggerInit=[525 437 675 493]  TopName=xmin_low  DataTypeOut=single  BankNumber=0  PreOverlay=false  PostOverlay=false  Role=Automatic
      settings: SourceProductName=Bose Talaria
  xmin TuneVar : TuneVar/TuneVar  TuneName=XMin  SpecifyMaxSize=off  VariableDim=2 (Column)  MaxSize=[1 1]  TunabilityNumber=1  MinValue=[]  MaxValue=[]  TriggerInit=[20 230 190 280]  MaskValue=Config.DefaultXmin
      settings: SourceProductName=Bose Talaria
  xmin TuneVar1 : TuneVar/TuneVar  TuneName=XMinLow  SpecifyMaxSize=off  VariableDim=2 (Column)  MaxSize=[1 1]  TunabilityNumber=1  MinValue=[]  MaxValue=[]  TriggerInit=[20 570 190 620]  MaskValue=Config.DefaultXminLow
      settings: SourceProductName=Bose Talaria
  ymax TuneVar : TuneVar/TuneVar  TuneName=YMax  SpecifyMaxSize=off  VariableDim=2 (Column)  MaxSize=[1 1]  TunabilityNumber=1  MinValue=[]  MaxValue=[]  TriggerInit=[20 120 190 170]  MaskValue=Config.DefaultYmax
      settings: SourceProductName=Bose Talaria
  ymax TuneVar1 : TuneVar/TuneVar  TuneName=YMaxLow  SpecifyMaxSize=off  VariableDim=2 (Column)  MaxSize=[1 1]  TunabilityNumber=1  MinValue=[]  MaxValue=[]  TriggerInit=[20 460 190 510]  MaskValue=Config.DefaultYmaxLow
      settings: SourceProductName=Bose Talaria
  wires:
  translation1/2(xmax_top) -> xmax TOP1/1
  translation1/3(p2) -> p2 TOP1/1
  translation1/1(xmin_top) -> xmin TOP1/1
  xmin TuneVar1/1 -> translation1/2(xmin_tune)  "XMinLow"
  ymax TuneVar1/1 -> translation1/1(ymax_tune)  "YMaxLow"
  TranslateTrigger1/1 -> translation1/Trigger
  TranslateTrigger/1 -> translation/Trigger
  xmin TuneVar/1 -> translation/2(xmin_tune)  "XMin"
  ymax TuneVar/1 -> translation/1(ymax_tune)  "YMax"
  translation/3(p2) -> p2 TOP/1
  translation/2(xmax_top) -> xmax TOP/1
  translation/1(xmin_top) -> xmin TOP/1

== system Model_TranslationEngine64/TestRouter/ASDRouter/InnerLink/AuxChannel_with_MATLAB_function ==
  TuneTOP_enable_aux_flag : Subsystem  mask(Talaria Trivial Tune TOP){TriggerInit=[-445 144 -315 176], TopName=EnableAux, TuneName=EnableAux, DataTypeOut=int32, MaskValue=Config.EnableAux, TunabilityNumber=1, MinValue=[], MaxValue=[], BankNumber=0, PreOverlay=false, PostOverlay=false, UseSameName=on}
      mask prompts: TriggerInit "Hidden: MoveFcn redraw"; TopName "Name:"; TuneName "Name of TuneVar:"; DataTypeOut "Data type:"; MaskValue "Default Value:"; TunabilityNumber "Tunability:"; MinValue "Min Value:"; MaxValue "Max Value:"; BankNumber "Target memory bank number:"; PreOverlay "Requires pre-overlay action:"; PostOverlay "Requires post-overlay action:"; UseSameName "Use same name for tune variable and TOP"
      mask help: The TuneTOP block encapsultes a Target Overlay Parameter, a Tune Variable, and a Trivial Translation between them.
      mask init:
      | [ok,activeTopPath,activeTunePath] = TuneTOP_Mask.Init(gcbh);
      settings: MoveFcn=TuneTOP_Mask.CB_TriggerInit(gcbh);
      mask Callback TriggerInit: TuneTOP_Mask.CB_TriggerInit(gcbh);
      mask TypeOptions TopName: TOP/TopName
      mask TypeOptions TuneName: Tune Variable/TuneName
      mask TypeOptions DataTypeOut: TOP/DataTypeOut
      mask TypeOptions MaskValue: Tune Variable/MaskValue
      mask TypeOptions TunabilityNumber: Tune Variable/TunabilityNumber
      mask Callback TunabilityNumber: TuneVarMask.CB_TunabilityNumber(gcbh);
      mask TypeOptions MinValue: Tune Variable/MinValue
      mask TypeOptions MaxValue: Tune Variable/MaxValue
      mask TypeOptions BankNumber: TOP/BankNumber
      mask TypeOptions PreOverlay: TOP/PreOverlay
      mask TypeOptions PostOverlay: TOP/PostOverlay
      mask Callback UseSameName: TuneTOP_Mask.CB_UseSameName(gcbh);
      mask DialogControl toolPanel Prompt: Tuning Tool Hints
      mask DialogControl DescriptionGroup Prompt: Description
      mask DialogControl EditDescription Prompt: Edit Description
      mask DialogControl EditDescription Callback: TuneTOP_Mask.CB_EditDescription(gcbh);
      mask DialogControl TunabilityText Prompt: Easy: Changes nearly every tuning.
      mask DialogControl AdvancedPanel Prompt: Advanced
      mask DialogControl ConvertToFullTranslation Prompt: Irreversible conversion to full translation
      mask DialogControl ConvertToFullTranslation Callback: TuneTOP_Mask.CB_ConvertToFullTranslation(gcbh);
      mask DialogControl ErrorContainer Prompt: Error Messages
      mask DialogControl ErrorText Prompt: Default value cannot be empty. Tune variables must have non-zero dimensions.
      mask Display:
      | % retrieve icon definition
      | [path,w,h] = TuneTOP_Mask.Icon();
      | 
      | % retrieve the block's pixel size
      | pos = get(gcbh,'position');
      | bw = pos(3) - pos(1);
      | bh = pos(4) - pos(2);
      | 
      | % draw centered icon
      | xAdj = bw/2 - w/2 + 5;
      | yAdj = bh/2 - h/2 + 4;
      | for i=1:length(path)
      | 	patch(path(i).x+xAdj, path(i).y+yAdj, path(i).rgb);
      | end
      | 
      | % show the top name or an X
      | if (exist('ok','var') && ok)
      | 	text(bw*0.5, bh*0.2, activeTopPath, 'horizontalAlignment', 'center');
      | 	patch(0,0,[1 1 1]);
      | 	patch(bw,bh,[1 1 1]);
      | else
      | 	tx=bw*0.03;
      | 	ty=bh*0.03;
      | 	patch([0 tx bw bw-tx], [ty 0 bh-ty bh], [1 0 0]);
      | 	patch([0 bw-tx bw tx], [bh-ty 0 ty bh], [1 0 0]);
      | end

== system Model_TranslationEngine64/TestRouter/ASDRouter/InnerLink/MainChannelSystem ==
  TuneTOP_pmain_select : Subsystem  mask(Talaria Trivial Tune TOP){TriggerInit=[-390 156 -225 204], TopName=MainSelect, TuneName=MainSelect, DataTypeOut=int32, MaskValue=Config.MainSelect, TunabilityNumber=1, MinValue=[], MaxValue=[], BankNumber=0, PreOverlay=false, PostOverlay=false, UseSameName=on}
      mask prompts: TriggerInit "Hidden: MoveFcn redraw"; TopName "Name:"; TuneName "Name of TuneVar:"; DataTypeOut "Data type:"; MaskValue "Default Value:"; TunabilityNumber "Tunability:"; MinValue "Min Value:"; MaxValue "Max Value:"; BankNumber "Target memory bank number:"; PreOverlay "Requires pre-overlay action:"; PostOverlay "Requires post-overlay action:"; UseSameName "Use same name for tune variable and TOP"
      mask help: The TuneTOP block encapsultes a Target Overlay Parameter, a Tune Variable, and a Trivial Translation between them.
      mask init:
      | [ok,activeTopPath,activeTunePath] = TuneTOP_Mask.Init(gcbh);
      settings: MoveFcn=TuneTOP_Mask.CB_TriggerInit(gcbh);
      mask Callback TriggerInit: TuneTOP_Mask.CB_TriggerInit(gcbh);
      mask TypeOptions TopName: TOP/TopName
      mask TypeOptions TuneName: Tune Variable/TuneName
      mask TypeOptions DataTypeOut: TOP/DataTypeOut
      mask TypeOptions MaskValue: Tune Variable/MaskValue
      mask TypeOptions TunabilityNumber: Tune Variable/TunabilityNumber
      mask Callback TunabilityNumber: TuneVarMask.CB_TunabilityNumber(gcbh);
      mask TypeOptions MinValue: Tune Variable/MinValue
      mask TypeOptions MaxValue: Tune Variable/MaxValue
      mask TypeOptions BankNumber: TOP/BankNumber
      mask TypeOptions PreOverlay: TOP/PreOverlay
      mask TypeOptions PostOverlay: TOP/PostOverlay
      mask Callback UseSameName: TuneTOP_Mask.CB_UseSameName(gcbh);
      mask DialogControl toolPanel Prompt: Tuning Tool Hints
      mask DialogControl DescriptionGroup Prompt: Description
      mask DialogControl EditDescription Prompt: Edit Description
      mask DialogControl EditDescription Callback: TuneTOP_Mask.CB_EditDescription(gcbh);
      mask DialogControl TunabilityText Prompt: Easy: Changes nearly every tuning.
      mask DialogControl AdvancedPanel Prompt: Advanced
      mask DialogControl ConvertToFullTranslation Prompt: Irreversible conversion to full translation
      mask DialogControl ConvertToFullTranslation Callback: TuneTOP_Mask.CB_ConvertToFullTranslation(gcbh);
      mask DialogControl ErrorContainer Prompt: Error Messages
      mask DialogControl ErrorText Prompt: Default value cannot be empty. Tune variables must have non-zero dimensions.
      mask Display:
      | % retrieve icon definition
      | [path,w,h] = TuneTOP_Mask.Icon();
      | 
      | % retrieve the block's pixel size
      | pos = get(gcbh,'position');
      | bw = pos(3) - pos(1);
      | bh = pos(4) - pos(2);
      | 
      | % draw centered icon
      | xAdj = bw/2 - w/2 + 5;
      | yAdj = bh/2 - h/2 + 4;
      | for i=1:length(path)
      | 	patch(path(i).x+xAdj, path(i).y+yAdj, path(i).rgb);
      | end
      | 
      | % show the top name or an X
      | if (exist('ok','var') && ok)
      | 	text(bw*0.5, bh*0.2, activeTopPath, 'horizontalAlignment', 'center');
      | 	patch(0,0,[1 1 1]);
      | 	patch(bw,bh,[1 1 1]);
      | else
      | 	tx=bw*0.03;
      | 	ty=bh*0.03;
      | 	patch([0 tx bw bw-tx], [ty 0 bh-ty bh], [1 0 0]);
      | 	patch([0 bw-tx bw tx], [bh-ty 0 ty bh], [1 0 0]);
      | end

== system Model_TranslationEngine64/ModelPreAmp/DecRate/AudioPilot35/Audiopilot_3_5/ConfigurationRtcInputs ==
  note: Downgrade Flag
  note: HVAC
  note: Speed
  note: Mute
  AudiopilotTwoDowngrade : Subsystem  mask(Talaria Trivial Tune TOP){TriggerInit=[1655 1312 1805 1368], TopName=TwoDowngrade, TuneName=TwoDowngrade, DataTypeOut=uint32, MaskValue=0, TunabilityNumber=1, MinValue=[], MaxValue=[], BankNumber=0, PreOverlay=false, PostOverlay=false, UseSameName=on}
      mask prompts: TriggerInit "Hidden: MoveFcn redraw"; TopName "Name:"; TuneName "Name of TuneVar:"; DataTypeOut "Data type:"; MaskValue "Default Value:"; TunabilityNumber "Tunability:"; MinValue "Min Value:"; MaxValue "Max Value:"; BankNumber "Target memory bank number:"; PreOverlay "Requires pre-overlay action:"; PostOverlay "Requires post-overlay action:"; UseSameName "Use same name for tune variable and TOP"
      mask help: The TuneTOP block encapsultes a Target Overlay Parameter, a Tune Variable, and a Trivial Translation between them.
      mask init:
      | [ok,activeTopPath,activeTunePath] = TuneTOP_Mask.Init(gcbh);
      settings: MoveFcn=TuneTOP_Mask.CB_TriggerInit(gcbh);
      mask Callback TriggerInit: TuneTOP_Mask.CB_TriggerInit(gcbh);
      mask TypeOptions TopName: TOP/TopName
      mask TypeOptions TuneName: Tune Variable/TuneName
      mask TypeOptions DataTypeOut: TOP/DataTypeOut
      mask TypeOptions MaskValue: Tune Variable/MaskValue
      mask TypeOptions TunabilityNumber: Tune Variable/TunabilityNumber
      mask Callback TunabilityNumber: TuneVarMask.CB_TunabilityNumber(gcbh);
      mask TypeOptions MinValue: Tune Variable/MinValue
      mask TypeOptions MaxValue: Tune Variable/MaxValue
      mask TypeOptions BankNumber: TOP/BankNumber
      mask TypeOptions PreOverlay: TOP/PreOverlay
      mask TypeOptions PostOverlay: TOP/PostOverlay
      mask Callback UseSameName: TuneTOP_Mask.CB_UseSameName(gcbh);
      mask DialogControl toolPanel Prompt: Tuning Tool Hints
      mask DialogControl DescriptionGroup Prompt: Description
      mask DialogControl EditDescription Prompt: Edit Description
      mask DialogControl EditDescription Callback: TuneTOP_Mask.CB_EditDescription(gcbh);
      mask DialogControl TunabilityText Prompt: Easy: Changes nearly every tuning.
      mask DialogControl AdvancedPanel Prompt: Advanced
      mask DialogControl ConvertToFullTranslation Prompt: Irreversible conversion to full translation
      mask DialogControl ConvertToFullTranslation Callback: TuneTOP_Mask.CB_ConvertToFullTranslation(gcbh);
      mask DialogControl ErrorContainer Prompt: Error Messages
      mask DialogControl ErrorText Prompt: No overlay group found. Declare one in a FeaturePath.
      mask Display:
      | % retrieve icon definition
      | [path,w,h] = TuneTOP_Mask.Icon();
      | 
      | % retrieve the block's pixel size
      | pos = get(gcbh,'position');
      | bw = pos(3) - pos(1);
      | bh = pos(4) - pos(2);
      | 
      | % draw centered icon
      | xAdj = bw/2 - w/2 + 5;
      | yAdj = bh/2 - h/2 + 4;
      | for i=1:length(path)
      | 	patch(path(i).x+xAdj, path(i).y+yAdj, path(i).rgb);
      | end
      | 
      | % show the top name or an X
      | if (exist('ok','var') && ok)
      | 	text(bw*0.5, bh*0.2, activeTopPath, 'horizontalAlignment', 'center');
      | 	patch(0,0,[1 1 1]);
      | 	patch(bw,bh,[1 1 1]);
      | else
      | 	tx=bw*0.03;
      | 	ty=bh*0.03;
      | 	patch([0 tx bw bw-tx], [ty 0 bh-ty bh], [1 0 0]);
      | 	patch([0 bw-tx bw tx], [bh-ty 0 ty bh], [1 0 0]);
      | end
  Hvac : Subsystem  mask(AudioPilot - HVAC Table){Config=Config.HVAC}
      mask prompts: Config "HVACConfig"
      mask help: This block implements the table lookup for the HVAC index. It has 16 entries and returns the HVAC level in dBSPL.
      mask init:
      | blkh = gcbh;
      | 
      | Config = BTConfig.Assert(blkh,Config);
      | Config.Validate();
      | 
      | MaskHvacTableSize = Config.HVACTableSize;
      mask Help:
      | This block implements the table lookup for the HVAC index.  It has 16 entries and returns the HVAC level in dBSPL.
      | 
      | Arguments for this block:
      | 
      | Configuration
      | The block can be configured using an object of class, HVACConfig.  If the "use Default Configuration Only" box is checked, then this option is disabled.
      mask DialogControl BTC Prompt: Build Time Configuration
      mask DialogControl Config Tooltip: The configuration has to be an object of the class, HVACConfig.

== system Model_TranslationEngine64/ModelPreAmp/DecRate/AudioPilot35/Audiopilot_3_5/GainApplication ==
  note: Gain Application
  Compensation : Subsystem

== system Model_TranslationEngine64/ModelPreAmp/DecRate/AudioPilot35/Audiopilot_3_5/GainCalculation ==
  note: Gain Calculation
  BoostMapAdjustment : Subsystem
  Boosts : Subsystem
  RampedEnable : Subsystem

== system Model_TranslationEngine64/ModelPreAmp/DecRate/AudioPilot35/Audiopilot_3_5/NoiseEstimationVariant ==
  RegularNoiseEstimation : Subsystem  VariantControl=Regular
  SpeedOnly : Subsystem  VariantControl=Speed Only  mask(AudioPilot - Speed Only Noise Estimation){Config=Config.SpeedOnly}
      mask prompts: Config "SpeedOnlyConfig"
      mask help: This block implements the speed only variant for noise estimation
      mask init:
      | blkh = gcbh;
      | 
      | Config = BTConfig.Assert(blkh,Config);
      | Config.Validate();
      | 
      | SampleRate = Config.SampleRateHz;
      | DecRate = Config.DecRateHz;
      mask Help:
      | This block implements the speed only variant for noise estimation.
      | 
      | Arguments for this block:
      | 
      | Configuration
      | The block can be configured using an object of class, SpeedOnlyConfig.  If the "use Default Configuration Only" box is checked, then this option is disabled.
      | 
      | Sample Rate
      | This is the sample rate of the input audio streams, typically 44100 Hz or 48 kHz.
      mask DialogControl BTC Prompt: Build Time Configuration
      mask DialogControl Config Tooltip: The configuration has to be an object of the class, SpeedOnlyConfig.

== system Model_TranslationEngine64/ModelPreAmp/DecRate/AudioPilot35/EntertainmentLevelDetection/AudiopilotLevelDetect ==
  AudiopilotLevelDetect : Subsystem

== system Model_TranslationEngine64/ModelPreAmp/DecRate/AudioPilot35/EntertainmentLevelDetection/DyneqLevelDetect ==
  DyneqLevelDetect : Subsystem
